simulink model "TestCase_Arch_RCCar_mapping"  (R2016b)
settings: Solver=FixedStepAuto  StartTime=0.0  StopTime=10.0  RelTol=1e-3
model workspace: external: MAT-File TestCase_Arch_RCCar_mapping.mat (data not in the file)
libraries: libTLAsserts x4, libAsserts x2
settings Model: Creator=NEATdemo  LastModifiedBy=NEATdemo

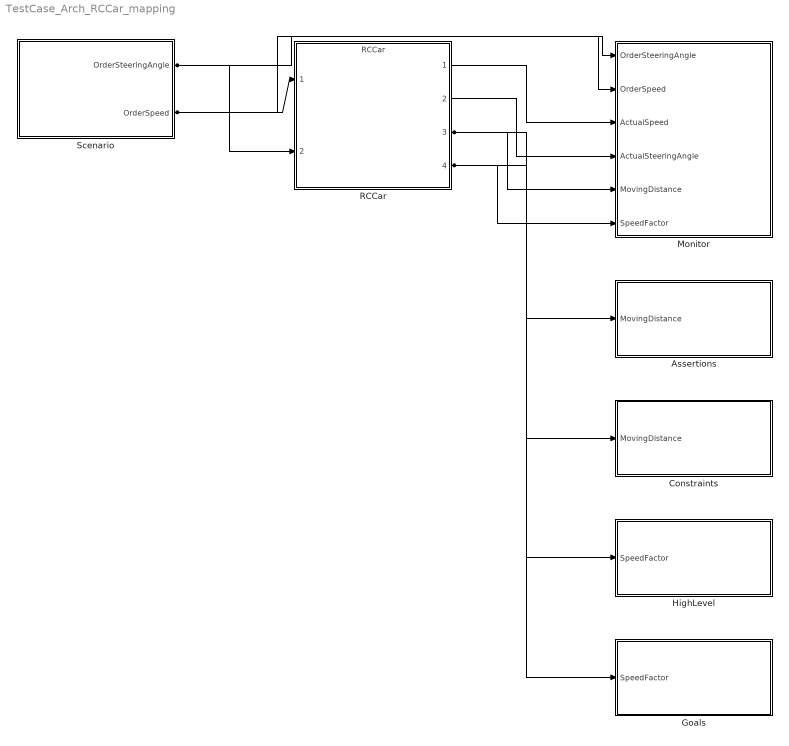
== system TestCase_Arch_RCCar_mapping ==
  Assertions : Subsystem
  Constraints : Subsystem
  Goals : Subsystem
  HighLevel : Subsystem
  Monitor : Subsystem
  RCCar : ModelReference  ModelNameDialog=RCCar  SimulationMode=Normal  ModelReferenceVersion=1.21
  Scenario : Subsystem
  wires:
  Scenario/1(OrderSteeringAngle) -> RCCar/2, Monitor/1(OrderSteeringAngle)
  Scenario/2(OrderSpeed) -> RCCar/1, Monitor/2(OrderSpeed)
  RCCar/1 -> Monitor/3(ActualSpeed)
  RCCar/2 -> Monitor/4(ActualSteeringAngle)
  RCCar/3 -> Monitor/5(MovingDistance), Assertions/1(MovingDistance), Constraints/1(MovingDistance)
  RCCar/4 -> Monitor/6(SpeedFactor), HighLevel/1(SpeedFactor), Goals/1(SpeedFactor)

== system TestCase_Arch_RCCar_mapping/Assertions ==
  MovingDistance : Inport
  assert_1 : Subsystem
  simout_1 : ToFile  Filename=assert_1.mat  MatrixName=assert_1  SaveFormat=Timeseries
  wires:
  MovingDistance/1 -> assert_1/1(MovingDistance)
  assert_1/1(assert_1_FAILED) -> simout_1/1

== system TestCase_Arch_RCCar_mapping/Constraints ==
  MovingDistance : Inport
  const_1 : Subsystem
  simout_1 : ToFile  Filename=const_1.mat  MatrixName=const_1  SaveFormat=Timeseries
  wires:
  MovingDistance/1 -> const_1/1(MovingDistance)
  const_1/1(const_1_FAILED) -> simout_1/1

== system TestCase_Arch_RCCar_mapping/Goals ==
  SpeedFactor : Inport
  goals_1 : Subsystem
  simout_1 : ToFile  Filename=goals_1.mat  MatrixName=goals_1  SaveFormat=Timeseries
  wires:
  SpeedFactor/1 -> goals_1/1(SpeedFactor)
  goals_1/1(goals_1_VAL) -> simout_1/1

== system TestCase_Arch_RCCar_mapping/HighLevel ==
  SpeedFactor : Inport
  highlevel_1 : Subsystem
  simout_1 : ToFile  Filename=highlevel_1.mat  MatrixName=highlevel_1  SaveFormat=Timeseries
  wires:
  SpeedFactor/1 -> highlevel_1/1(SpeedFactor)
  highlevel_1/1(highlevel_1_FAILED) -> simout_1/1

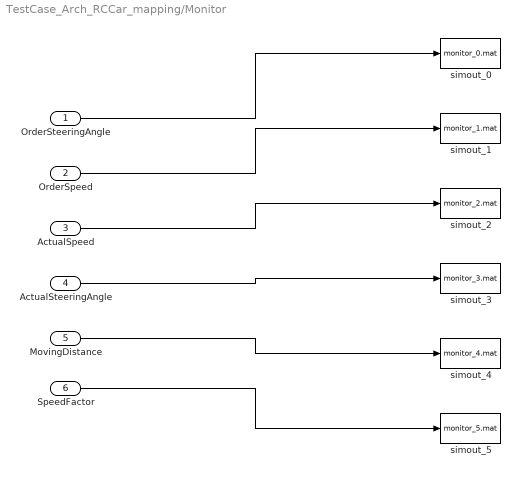
== system TestCase_Arch_RCCar_mapping/Monitor ==
  OrderSteeringAngle : Inport
  OrderSpeed : Inport  Port=2
  ActualSpeed : Inport  Port=3
  ActualSteeringAngle : Inport  Port=4
  MovingDistance : Inport  Port=5
  SpeedFactor : Inport  Port=6
  simout_0 : ToFile  Filename=monitor_0.mat  MatrixName=OrderSteeringAngle  SaveFormat=Timeseries
  simout_1 : ToFile  Filename=monitor_1.mat  MatrixName=OrderSpeed  SaveFormat=Timeseries
  simout_2 : ToFile  Filename=monitor_2.mat  MatrixName=ActualSpeed  SaveFormat=Timeseries
  simout_3 : ToFile  Filename=monitor_3.mat  MatrixName=ActualSteeringAngle  SaveFormat=Timeseries
  simout_4 : ToFile  Filename=monitor_4.mat  MatrixName=MovingDistance  SaveFormat=Timeseries
  simout_5 : ToFile  Filename=monitor_5.mat  MatrixName=SpeedFactor  SaveFormat=Timeseries
  wires:
  OrderSteeringAngle/1 -> simout_0/1
  OrderSpeed/1 -> simout_1/1
  ActualSpeed/1 -> simout_2/1
  ActualSteeringAngle/1 -> simout_3/1
  MovingDistance/1 -> simout_4/1
  SpeedFactor/1 -> simout_5/1

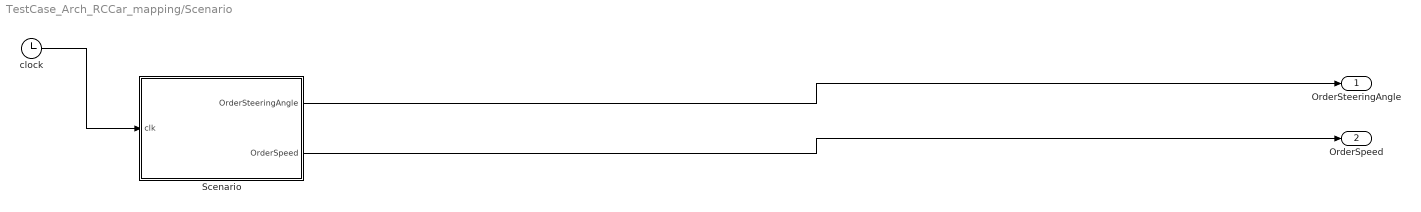
== system TestCase_Arch_RCCar_mapping/Scenario ==
  Scenario : Stateflow chart  TreatAsAtomicUnit=on
  clock : Clock
  OrderSteeringAngle : Outport
  OrderSpeed : Outport  Port=2
  wires:
  Scenario/1(OrderSteeringAngle) -> OrderSteeringAngle/1
  Scenario/2(OrderSpeed) -> OrderSpeed/1
  clock/1 -> Scenario/1(clk)

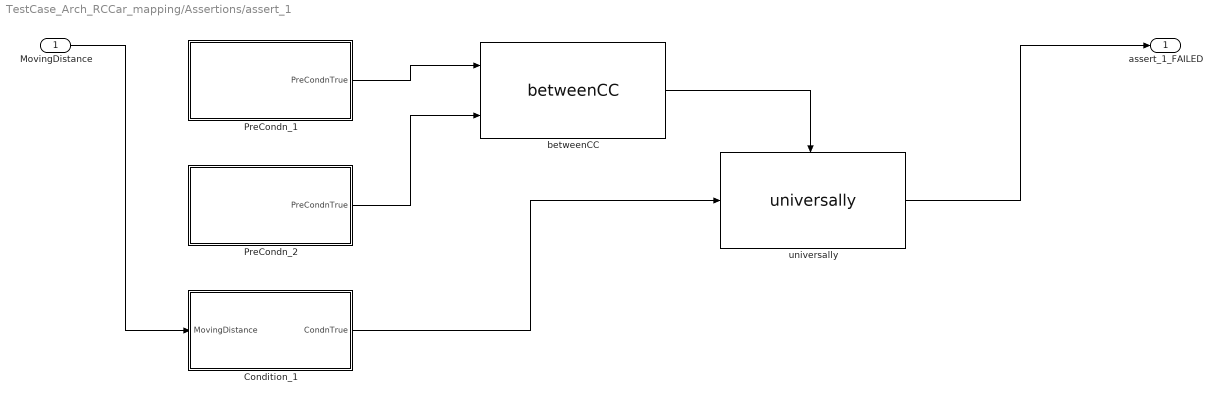
== system TestCase_Arch_RCCar_mapping/Assertions/assert_1 ==
  MovingDistance : Inport
  Condition_1 : Subsystem
  PreCondn_1 : Subsystem
  PreCondn_2 : Subsystem
  betweenCC : libTLAsserts/betweenCC
  universally : libTLAsserts/universally
  assert_1_FAILED : Outport
  wires:
  MovingDistance/1 -> Condition_1/1(MovingDistance)
  PreCondn_1/1(PreCondnTrue) -> betweenCC/1
  PreCondn_2/1(PreCondnTrue) -> betweenCC/2
  Condition_1/1(CondnTrue) -> universally/1
  betweenCC/1 -> universally/Enable
  universally/1 -> assert_1_FAILED/1

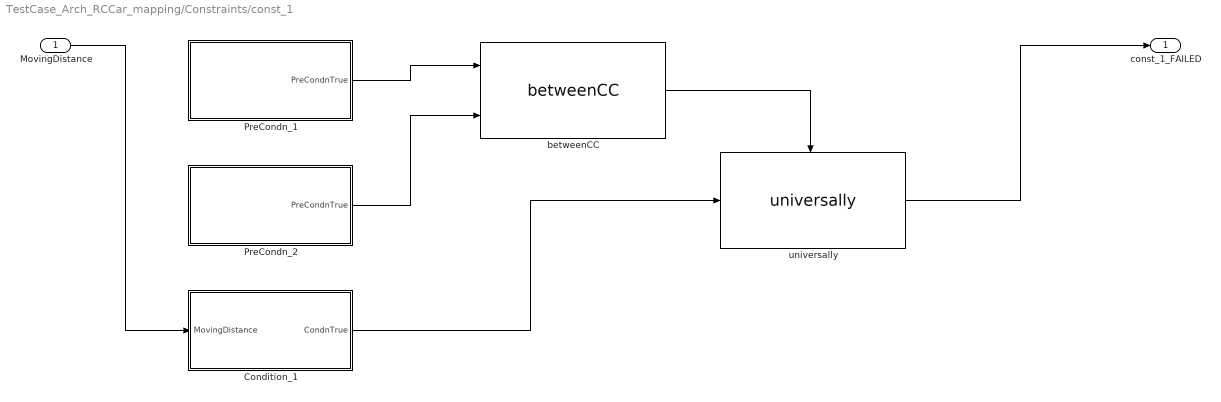
== system TestCase_Arch_RCCar_mapping/Constraints/const_1 ==
  MovingDistance : Inport
  Condition_1 : Subsystem
  PreCondn_1 : Subsystem
  PreCondn_2 : Subsystem
  betweenCC : libTLAsserts/betweenCC
  universally : libTLAsserts/universally
  const_1_FAILED : Outport
  wires:
  MovingDistance/1 -> Condition_1/1(MovingDistance)
  PreCondn_1/1(PreCondnTrue) -> betweenCC/1
  PreCondn_2/1(PreCondnTrue) -> betweenCC/2
  Condition_1/1(CondnTrue) -> universally/1
  betweenCC/1 -> universally/Enable
  universally/1 -> const_1_FAILED/1

== system TestCase_Arch_RCCar_mapping/Goals/goals_1 ==
  SpeedFactor : Inport
  goals_1_VAL : Outport
  wires:
  SpeedFactor/1 -> goals_1_VAL/1

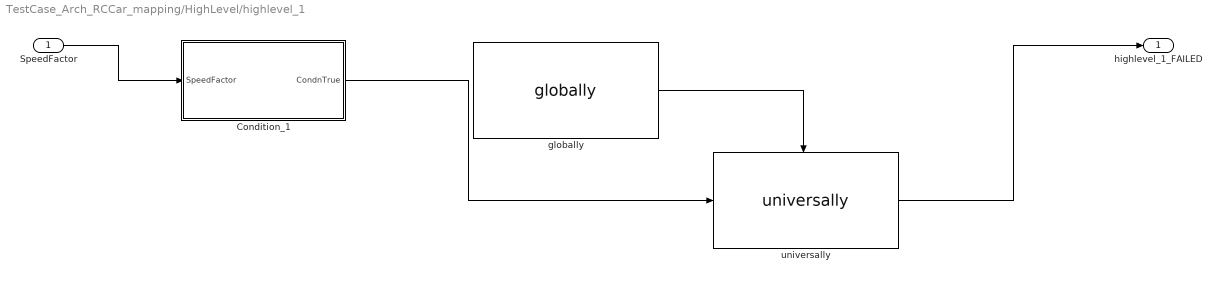
== system TestCase_Arch_RCCar_mapping/HighLevel/highlevel_1 ==
  SpeedFactor : Inport
  Condition_1 : Subsystem
  globally : libAsserts/globally
  universally : libAsserts/universally
  highlevel_1_FAILED : Outport
  wires:
  SpeedFactor/1 -> Condition_1/1(SpeedFactor)
  Condition_1/1(CondnTrue) -> universally/1
  universally/1 -> highlevel_1_FAILED/1
  globally/1 -> universally/Enable

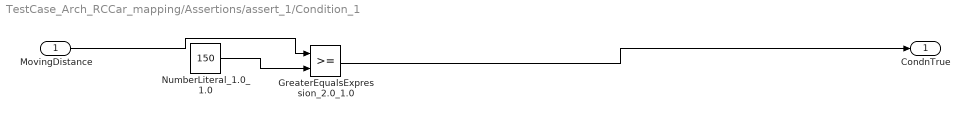
== system TestCase_Arch_RCCar_mapping/Assertions/assert_1/Condition_1 ==
  MovingDistance : Inport
  GreaterEqualsExpression_2.0_1.0 : RelationalOperator  OutDataTypeStr=boolean  RndMeth=Simplest
  NumberLiteral_1.0_1.0 : Constant  Value=150
  CondnTrue : Outport
  wires:
  MovingDistance/1 -> GreaterEqualsExpression_2.0_1.0/1
  NumberLiteral_1.0_1.0/1 -> GreaterEqualsExpression_2.0_1.0/2
  GreaterEqualsExpression_2.0_1.0/1 -> CondnTrue/1

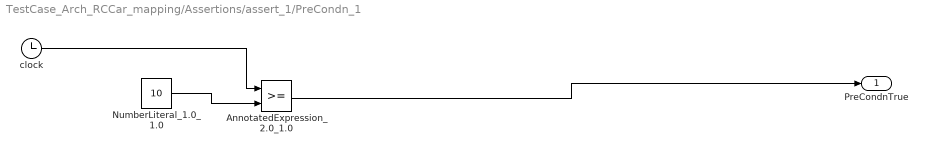
== system TestCase_Arch_RCCar_mapping/Assertions/assert_1/PreCondn_1 ==
  AnnotatedExpression_2.0_1.0 : RelationalOperator  OutDataTypeStr=boolean  RndMeth=Simplest
  NumberLiteral_1.0_1.0 : Constant  Value=10
  clock : Clock
  PreCondnTrue : Outport
  wires:
  clock/1 -> AnnotatedExpression_2.0_1.0/1
  NumberLiteral_1.0_1.0/1 -> AnnotatedExpression_2.0_1.0/2
  AnnotatedExpression_2.0_1.0/1 -> PreCondnTrue/1

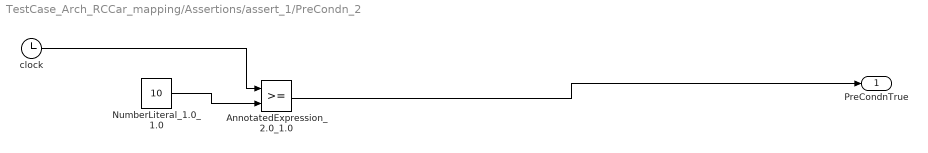
== system TestCase_Arch_RCCar_mapping/Assertions/assert_1/PreCondn_2 ==
  AnnotatedExpression_2.0_1.0 : RelationalOperator  OutDataTypeStr=boolean  RndMeth=Simplest
  NumberLiteral_1.0_1.0 : Constant  Value=10
  clock : Clock
  PreCondnTrue : Outport
  wires:
  clock/1 -> AnnotatedExpression_2.0_1.0/1
  NumberLiteral_1.0_1.0/1 -> AnnotatedExpression_2.0_1.0/2
  AnnotatedExpression_2.0_1.0/1 -> PreCondnTrue/1

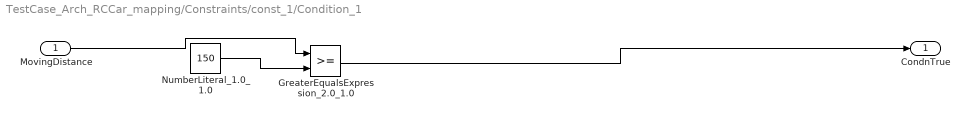
== system TestCase_Arch_RCCar_mapping/Constraints/const_1/Condition_1 ==
  MovingDistance : Inport
  GreaterEqualsExpression_2.0_1.0 : RelationalOperator  OutDataTypeStr=boolean  RndMeth=Simplest
  NumberLiteral_1.0_1.0 : Constant  Value=150
  CondnTrue : Outport
  wires:
  MovingDistance/1 -> GreaterEqualsExpression_2.0_1.0/1
  NumberLiteral_1.0_1.0/1 -> GreaterEqualsExpression_2.0_1.0/2
  GreaterEqualsExpression_2.0_1.0/1 -> CondnTrue/1

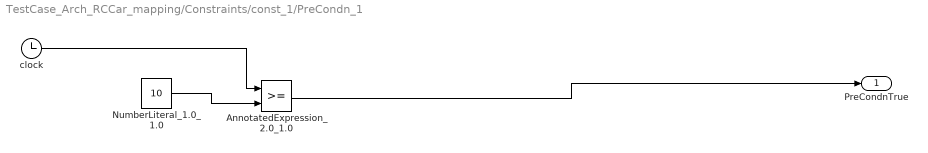
== system TestCase_Arch_RCCar_mapping/Constraints/const_1/PreCondn_1 ==
  AnnotatedExpression_2.0_1.0 : RelationalOperator  OutDataTypeStr=boolean  RndMeth=Simplest
  NumberLiteral_1.0_1.0 : Constant  Value=10
  clock : Clock
  PreCondnTrue : Outport
  wires:
  clock/1 -> AnnotatedExpression_2.0_1.0/1
  NumberLiteral_1.0_1.0/1 -> AnnotatedExpression_2.0_1.0/2
  AnnotatedExpression_2.0_1.0/1 -> PreCondnTrue/1

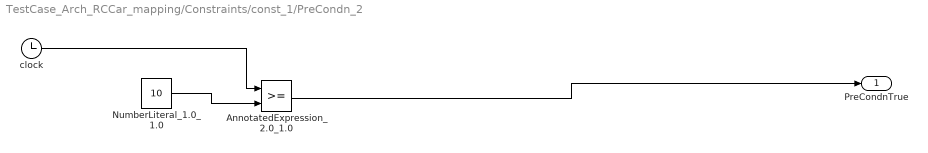
== system TestCase_Arch_RCCar_mapping/Constraints/const_1/PreCondn_2 ==
  AnnotatedExpression_2.0_1.0 : RelationalOperator  OutDataTypeStr=boolean  RndMeth=Simplest
  NumberLiteral_1.0_1.0 : Constant  Value=10
  clock : Clock
  PreCondnTrue : Outport
  wires:
  clock/1 -> AnnotatedExpression_2.0_1.0/1
  NumberLiteral_1.0_1.0/1 -> AnnotatedExpression_2.0_1.0/2
  AnnotatedExpression_2.0_1.0/1 -> PreCondnTrue/1

== system TestCase_Arch_RCCar_mapping/HighLevel/highlevel_1/Condition_1 ==
  SpeedFactor : Inport
  GreaterEqualsExpression_2.0_1.0 : RelationalOperator  OutDataTypeStr=boolean  RndMeth=Simplest
  NumberLiteral_1.0_1.0 : Constant  Value=0.5
  CondnTrue : Outport
  wires:
  SpeedFactor/1 -> GreaterEqualsExpression_2.0_1.0/1
  NumberLiteral_1.0_1.0/1 -> GreaterEqualsExpression_2.0_1.0/2
  GreaterEqualsExpression_2.0_1.0/1 -> CondnTrue/1

== stateflow chart TestCase_Arch_RCCar_mapping/Scenario/Scenario ==
  state Act_Controller [parallel]
    settings: executionOrder=1
    state Act_Controller_Step1
      entry: OrderSteeringAngle = 0;
      entry: OrderSpeed = 30;
      entry: Act_Controller_Step1_stpClk = clk;
    state Act_Controller_Step2
      entry: OrderSteeringAngle = -2;
      entry: Act_Controller_Step2_stpClk = clk;
    state Act_Controller_Step3
      entry: OrderSteeringAngle = 2;
      entry: Act_Controller_Step3_stpClk = clk;
    state Act_Controller_Step4
      entry: Act_Controller_Step4_stpClk = clk;
    (default) -> Act_Controller_Step1
    Act_Controller_Step1 -> Act_Controller_Step2 : [clk - Act_Controller_Step1_stpClk >= 4]
    Act_Controller_Step2 -> Act_Controller_Step3 : [clk - Act_Controller_Step2_stpClk >= 5]
    Act_Controller_Step3 -> Act_Controller_Step4 : [clk - Act_Controller_Step3_stpClk >= 7]
  state Act_Car [parallel]
    settings: executionOrder=2
    state Act_Car_Step1
      entry: Act_Car_Step1_stpClk = clk;
    (default) -> Act_Car_Step1
  data: clk input; OrderSteeringAngle output; OrderSpeed output; Act_Controller_Step1_stpClk local; Act_Controller_Step2_stpClk local; Act_Controller_Step3_stpClk local; Act_Controller_Step4_stpClk local; Act_Car_Step1_stpClk local
